simulink model "QASKTransmitter"  (R2019b)
settings: Solver=VariableStepAuto  StartTime=0.0  StopTime=5  RelTol=1e-3
settings Model: Creator=z3454314  LastModifiedBy=z3454314

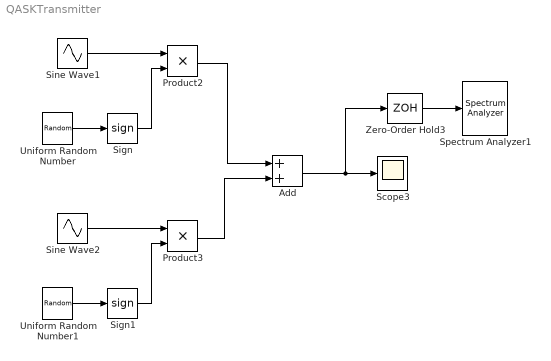
== system QASKTransmitter ==
  Add : Sum
  Product2 : Product
  Product3 : Product
  Scope3 : Scope
  Sign : Signum
  Sign1 : Signum
  Sine Wave1 : Sin  Frequency=8000*2*pi  SampleTime=0
  Sine Wave2 : Sin  Frequency=8000*2*pi  Phase=pi/2  SampleTime=0
  Spectrum Analyzer1 : SpectrumAnalyzer
  Uniform Random Number : UniformRandomNumber  SampleTime=1/2000
  Uniform Random Number1 : UniformRandomNumber  Seed=1  SampleTime=1/2000
  Zero-Order Hold3 : ZeroOrderHold  SampleTime=1/500e3
  wires:
  Uniform Random Number/1 -> Sign/1
  Sign/1 -> Product2/2
  Sine Wave1/1 -> Product2/1
  Sine Wave2/1 -> Product3/1
  Product3/1 -> Add/2
  Sign1/1 -> Product3/2
  Uniform Random Number1/1 -> Sign1/1
  Product2/1 -> Add/1
  Add/1 -> Zero-Order Hold3/1, Scope3/1
  Zero-Order Hold3/1 -> Spectrum Analyzer1/1
